simulink model "main"  (R2021a)
settings: Solver=FixedStepDiscrete  StartTime=0  StopTime=20  FixedStep=0.1  RelTol=1e-3
PreLoadFcn:
  | preloadFcn
values from neighbouring files (symbols this model uses):
  egoTargetSpd_kph = 60    [preloadFcn.m]
  iniEgoHeading = egoInfo(1,3)    [preloadFcn.m]
  iniEgoPos = egoInfo(1,1:2)    [preloadFcn.m]
  iniEgoSpd = egoInfo(1,4:5)    [preloadFcn.m]
  iniObsHeading1 = refInfo_obs1(1,3)    [preloadFcn.m]
  iniObsHeading2 = refInfo_obs2(1,3)    [preloadFcn.m]
  iniObsPos1 = refInfo_obs1(1,1:2)    [preloadFcn.m]
  iniObsPos2 = refInfo_obs2(1,1:2)    [preloadFcn.m]
  iniObsSpd1 = refInfo_obs1(1,4:5)    [preloadFcn.m]
  iniObsSpd2 = refInfo_obs2(1,4:5)    [preloadFcn.m]
  mu = [-2.06408447904 -1.49508472185]    [dataSet.mat]
  sig = [50.3880002876 29.2458553231]    [dataSet.mat]
undefined symbols (not defined in the file or in its folder): leftWaypoints, refInfo_obs1, refInfo_obs2, rightWaypoints
libraries: deeplib x2, fuzblock x1
(part 2 of 2)

== matlab function main/建立ST图 ==
  data: obsPos1 input; obsPos2 input; preTraj_real1 input; preTraj_real2 input; refPath input; obs_lb output; obs_ub output; cumLength input; obsZone1 output; obsZone2 output
function [obs_lb,obs_ub,obsZone1,obsZone2] = genST(obsPos1, obsPos2, preTraj_real1,preTraj_real2,refPath, cumLength)
%% 主程序
% 获取障碍车轨迹
obsPath1 = [obsPos1'; preTraj_real1];
obsPath2 = [obsPos2'; preTraj_real2];

% 初始化
ptNum = 81;
obs_lb = zeros(ptNum,3);
obs_ub =  zeros(ptNum,3);
obs_lb(:,1) = (0:0.1:8)';
obs_ub(:,1) = (0:0.1:8)';

% 映射第一个障碍车
[lb, ub] = getBound(refPath,obsPath1,ptNum,cumLength);
obs_lb(:,2) = lb;
obs_ub(:,2) = ub;

% 映射第二个障碍车
[lb, ub] = getBound(refPath,obsPath2,ptNum,cumLength);
obs_lb(:,3) = lb;
obs_ub(:,3) = ub;

% 获得ST图障碍区封闭边界（从障碍区下边界起始点开始逆时针，直到上边界起点），用于可视化画图
[obsZone1, obsZone2] = getObsZone(obs_lb,obs_ub);

end

%% 函数
% 交通车向本车参考路径的投影
function [lb, ub] = getBound(refPath,obsPath,ptNum,cumLength)
% 车辆参数
vehLength = 4.7;
vehWidth = 1.8;
vehHalfWidth = vehWidth/2;

lb = zeros(ptNum,1);
ub = zeros(ptNum,1);
for i = 1:ptNum-1
    % 车尾中心点位置和车辆航向角
    rearPosX = obsPath(i,1);
    rearPosY = obsPath(i,2);
    
    % 计算航向角
    diffX = obsPath(i+1,1) - obsPath(i,1);
    diffY =  obsPath(i+1,2) - obsPath(i,2);
    heading = atan2(diffY, diffX);
    
    % 根据车尾中心点位置和航向角计算车头中心点位置
    frontPosX = rearPosX + vehLength * cos(heading);
    frontPosY = rearPosY + vehLength * sin(heading);
    
    % 根据前后中心点、航向角计算目障碍车四个轮廓点位置（顺时针编号）
    % 每一行代表一个车辆一个角的纵向和横向位置
    VehPoints = zeros(4,2);
    VehPoints(1,1) = rearPosX - vehHalfWidth * sin(heading);
    VehPoints(1,2) = rearPosY + vehHalfWidth * cos(heading);
    VehPoints(2,1) = frontPosX - vehHalfWidth * sin(heading);
    VehPoints(2,2) = frontPosY + vehHalfWidth * cos(heading);
    VehPoints(3,1) = frontPosX + vehHalfWidth * sin(heading);
    VehPoints(3,2) = frontPosY - vehHalfWidth * cos(heading);
    VehPoints(4,1) = rearPosX + vehHalfWidth * sin(heading);
    VehPoints(4,2) = rearPosY - vehHalfWidth * cos(heading);
    
    % 依次计算四个点位置距离自车轨迹序列的最小距离的索引
    minDistTemp = zeros(1,4);
    minIndexTemp = zeros(1,4);
    for j = 1:4
        distX = refPath(1:30,1) - VehPoints(j,1);
        distY = refPath(1:30,2) - VehPoints(j,2);
        dist = sqrt((distX.^2 + distY.^2));
        [minDistTemp(j), minIndexTemp(j)] =  min(dist);
    end
    
    % 然后在四个距离中再次选择最小值，表征障碍车辆轮廓与本车轨迹的最小距离
    minDist = min(minDistTemp);
    
    % 若最小距离值小于阈值，表明障碍车在本时刻将会占据本车轨迹
    if minDist < 2.2
        % 计算minIndexTemp的最小索引和最大索引
        minIdx = min(minIndexTemp);
        maxIdx = max(minIndexTemp);
        
        % 然后获得S的下边界和上边界
        lb(i) = cumLength(minIdx);
        ub(i) = cumLength(maxIdx);
    else
        lb(i) = inf;
        ub(i) = -inf;
    end
end
lb(ptNum) = lb(ptNum-1);
ub(ptNum) = ub(ptNum-1);
end

% 获得ST图障碍区封闭边界
function [obsZone1, obsZone2] = getObsZone(obs_lb,obs_ub)
obsZone1 = zeros(160,2);
obsZone2 = zeros(160,2);

% 下边界
num1 = 0;
num2 = 0;
for i = 1:81
    t = (i-1)*0.1;
    if ~isinf(obs_lb(i,2))
        num1 = num1 + 1;
        obsZone1(num1,:) = [t,obs_lb(i,2)];
    end
    if ~isinf(obs_lb(i,3))
        num2 = num2 + 1;
        obsZone2(num2,:) = [t,obs_lb(i,3)];
    end
end

% 上边界
for i = 81:-1:1
    t = (i-1)*0.1;
    if ~isinf(obs_ub(i,2))
        num1 = num1 + 1;
        obsZone1(num1,:) = [t,obs_ub(i,2)];
    end
    if ~isinf(obs_ub(i,3))
        num2 = num2 + 1;
        obsZone2(num2,:) = [t,obs_ub(i,3)];
    end
end
end
